simulink model "Bilanciamento_MPC"  (R2026b)
settings: Solver=FixedStepDiscrete  StartTime=0  StopTime=sl.t_fine  FixedStep=sl.Ts_integrazione
PostLoadFcn:
  | addpath(genpath(fileparts(fileparts(get_param('Bilanciamento_MPC', 'FileName')))));
  | if ~evalin('base', 'exist(''sl'', ''var'')')
  |     assignin('base', 'sl', init_simulink());
  | end
InitFcn:
  | addpath(genpath(fileparts(fileparts(get_param('Bilanciamento_MPC', 'FileName')))));
  | if ~evalin('base', 'exist(''sl'', ''var'')')
  |     assignin('base', 'sl', init_simulink());
  | end
undefined symbols (not defined in the file or in its folder): sl
libraries: simulink x2
settings Model: Creator=Acer  LastModifiedBy=Acer

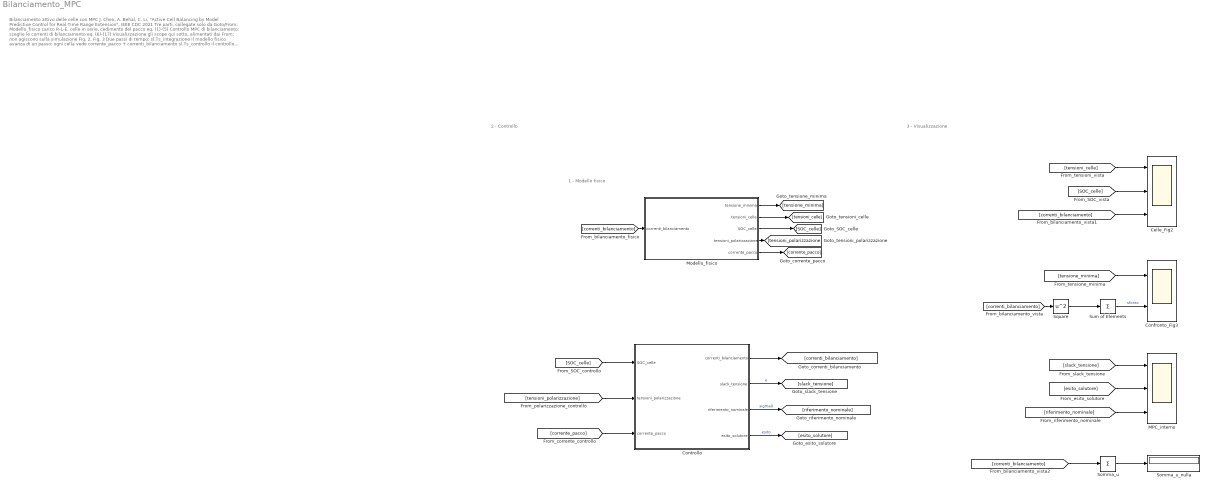
== system Bilanciamento_MPC ==
  note: Bilanciamento attivo delle celle con MPC
      | J. Chen, A. Behal, C. Li, "Active Cell Balancing by Model Predictive Control for Real Time Range Extension", IEEE CDC 2021
      |
      | Tre parti, collegate solo da Goto/From:
      |    Modello_fisico     carico R-L-E, celle in serie, cedimento del pacco             eq. (1)-(5)
      |    Controllo          MPC di bilanciamento: sceglie le correnti di bilanciamento    eq. (6)-(17)
      |    Visualizzazione    gli scope qui sotto, alimentati dai From: non agiscono sulla simulazione   Fig. 2, Fig. 3
      |
      | Due passi di tempo:
      |    sl.Ts_integrazione   il modello fisico avanza di un passo: ogni cella vede corrente_pacco + correnti_bilanciamento
      |    sl.Ts_controllo      il controllo campiona corrente_pacco, SOC_celle e tensioni_polarizzazione e sceglie correnti_bilanciamento,
      |                         che restano costanti fino al passo di controllo successivo
      | La simulazione si ferma quando una cella scende sotto y_min.
      |
      | Parametri nella struct 'sl' (avvio_simulink.m).  sl.tipo: 1 = J_t   2 = J_m   3 = J_Delta.  Confronto dei quattro casi: main_simulink.m
  note: 1 - Modello fisico
  note: 2 - Controllo
  note: 3 - Visualizzazione
  Celle_Fig2 : Scope  NumInputPorts=3
      settings: AttributesFormatString=Fig. 2: y, s, u  ActiveDisplayString=3  Title=Corrente di bilanciamento u^n [A]  ActiveDisplayYMinimum=-2.4917702044223984  ActiveDisplayYMaximum=2.42593183980159
  Confronto_Fig3 : Scope  NumInputPorts=2
      settings: AttributesFormatString=Fig. 3: min y, sforzo  Title=Sforzo di bilanciamento e_k = u_k'u_k [A^2]  ActiveDisplayYMinimum=0.52817346836693146  ActiveDisplayYMaximum=4.5629080222727767  DataLoggingVariableName=ScopeData2
  Controllo : Subsystem
      settings: AttributesFormatString=MPC: problema (6) risolto\ncome QP (Remark 3)
  MPC_interno : Scope  NumInputPorts=3
      settings: AttributesFormatString=slack e, esito, sigma0  ActiveDisplayString=3  Title=Riferimento della cella nominale sigma0, eq. (7): una linea per passo dell'orizzonte  ActiveDisplayYMinimum=-0.5240999999999999  ActiveDisplayYMaximum=4.7169
  Modello_fisico : Subsystem
      settings: AttributesFormatString=carico, celle, cedimento\neq. (1)-(5)
  Somma_u : Sum  Inputs=+
      settings: AttributesFormatString=eq. (6f)
  Somma_u_nulla : Display
      settings: AttributesFormatString=deve restare 0
  Square : Math  Operator=square
  Sum of Elements : Sum  Inputs=+
  wires:
  [correnti_bilanciamento] -> Square/1
  Square/1 -> Sum of Elements/1
  [correnti_bilanciamento] -> Somma_u/1
  [correnti_bilanciamento] -> Celle_Fig2/3
  [riferimento_nominale] -> MPC_interno/3
  [esito_solutore] -> MPC_interno/2
  [SOC_celle] -> Celle_Fig2/2
  [slack_tensione] -> MPC_interno/1
  [tensioni_celle] -> Celle_Fig2/1
  Sum of Elements/1 -> Confronto_Fig3/2  "sforzo"
  [tensione_minima] -> Confronto_Fig3/1
  Somma_u/1 -> Somma_u_nulla/1
  Controllo/4(esito_solutore) -> [esito_solutore]  "esito"
  Controllo/3(riferimento_nominale) -> [riferimento_nominale]  "sigma0"
  Controllo/2(slack_tensione) -> [slack_tensione]  "e"
  Controllo/1(correnti_bilanciamento) -> [correnti_bilanciamento]
  Modello_fisico/5(corrente_pacco) -> [corrente_pacco]
  Modello_fisico/4(tensioni_polarizzazione) -> [tensioni_polarizzazione]
  Modello_fisico/3(SOC_celle) -> [SOC_celle]
  Modello_fisico/2(tensioni_celle) -> [tensioni_celle]
  Modello_fisico/1(tensione_minima) -> [tensione_minima]
  [corrente_pacco] -> Controllo/3(corrente_pacco)
  [tensioni_polarizzazione] -> Controllo/2(tensioni_polarizzazione)
  [SOC_celle] -> Controllo/1(SOC_celle)
  [correnti_bilanciamento] -> Modello_fisico/1(correnti_bilanciamento)

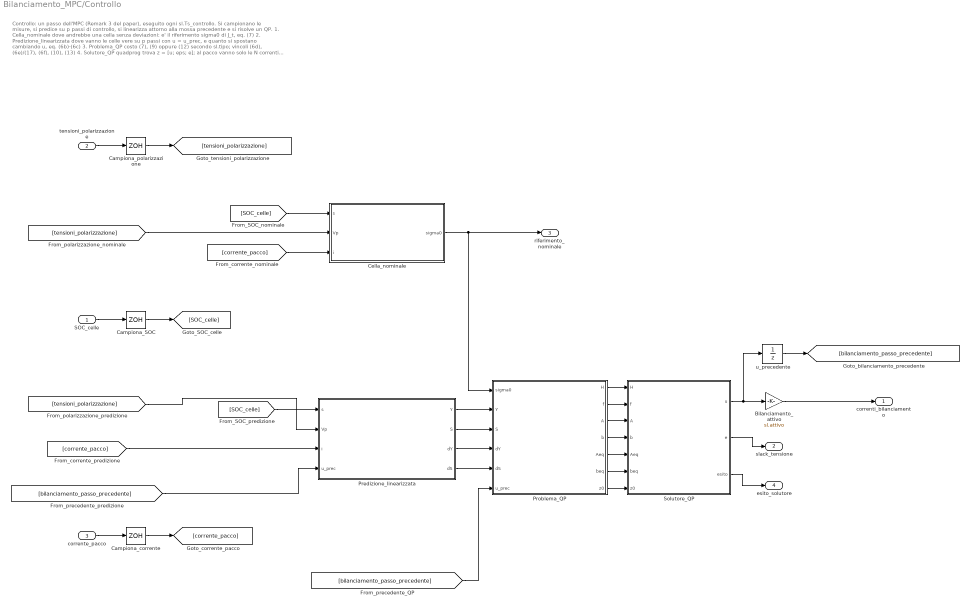
== system Bilanciamento_MPC/Controllo ==
  note: Controllo: un passo dell'MPC (Remark 3 del paper), eseguito ogni sl.Ts_controllo. Si campionano le misure, si predice su p passi di controllo,
      | si linearizza attorno alla mossa precedente e si risolve un QP.
      |
      | 1. Cella_nominale            dove andrebbe una cella senza deviazioni: e' il riferimento sigma0 di J_t, eq. (7)
      | 2. Predizione_linearizzata   dove vanno le celle vere su p passi con u = u_prec, e quanto si spostano cambiando u, eq. (6b)-(6c)
      | 3. Problema_QP               costo (7), (9) oppure (12) secondo sl.tipo; vincoli (6d), (6e)/(17), (6f), (10), (13)
      | 4. Solutore_QP               quadprog trova z = [u; eps; e]; al pacco vanno solo le N correnti u (orizzonte mobile)
      | 5. Bilanciamento_attivo      guadagno sl.attivo: con 0 il pacco lavora senza bilanciamento
      |
      | Doppio clic su un blocco per leggerne il codice; il calcolo vero e' nel file qp_*.m indicato nel commento.
  SOC_celle : Inport
  tensioni_polarizzazione : Inport  Port=2
  corrente_pacco : Inport  Port=3
  Bilanciamento_attivo : Gain  Gain=sl.attivo
      settings: AttributesFormatString=sl.attivo: 0 o 1
  Campiona_SOC : ZeroOrderHold  SampleTime=sl.Ts_controllo
      settings: AttributesFormatString=ogni Ts_controllo
  Campiona_corrente : ZeroOrderHold  SampleTime=sl.Ts_controllo
      settings: AttributesFormatString=ogni Ts_controllo
  Campiona_polarizzazione : ZeroOrderHold  SampleTime=sl.Ts_controllo
      settings: AttributesFormatString=ogni Ts_controllo
  Cella_nominale : MATLAB Function  TreatAsAtomicUnit=on
      settings: AttributesFormatString=eq. (7): riferimento sigma0
  Predizione_linearizzata : MATLAB Function  TreatAsAtomicUnit=on
      settings: AttributesFormatString=eq. (6b)-(6c), Remark 3
  Problema_QP : MATLAB Function  TreatAsAtomicUnit=on
      settings: AttributesFormatString=costo (7)/(9)/(12) e vincoli
  Solutore_QP : MATLAB Function  TreatAsAtomicUnit=on
      settings: AttributesFormatString=quadprog
  u_precedente : UnitDelay  InitialCondition=zeros(sl.N, 1)  SampleTime=sl.Ts_controllo
      settings: AttributesFormatString=u_(k-1)
  correnti_bilanciamento : Outport
  slack_tensione : Outport  Port=2
  riferimento_nominale : Outport  Port=3
  esito_solutore : Outport  Port=4
  wires:
  corrente_pacco/1 -> Campiona_corrente/1
  tensioni_polarizzazione/1 -> Campiona_polarizzazione/1
  SOC_celle/1 -> Campiona_SOC/1
  [corrente_pacco] -> Predizione_linearizzata/3(i)
  [tensioni_polarizzazione] -> Predizione_linearizzata/2(Vp)
  [SOC_celle] -> Predizione_linearizzata/1(s)
  [corrente_pacco] -> Cella_nominale/3(i)
  [tensioni_polarizzazione] -> Cella_nominale/2(Vp)
  [SOC_celle] -> Cella_nominale/1(s)
  Cella_nominale/1(sigma0) -> riferimento_nominale/1, Problema_QP/1(sigma0)
  Predizione_linearizzata/1(Y) -> Problema_QP/2(Y)
  Predizione_linearizzata/2(S) -> Problema_QP/3(S)
  Predizione_linearizzata/3(dY) -> Problema_QP/4(dY)
  Predizione_linearizzata/4(dS) -> Problema_QP/5(dS)
  Problema_QP/1(H) -> Solutore_QP/1(H)
  Problema_QP/2(f) -> Solutore_QP/2(f)
  Problema_QP/3(A) -> Solutore_QP/3(A)
  Problema_QP/4(b) -> Solutore_QP/4(b)
  Problema_QP/5(Aeq) -> Solutore_QP/5(Aeq)
  Problema_QP/6(beq) -> Solutore_QP/6(beq)
  Problema_QP/7(z0) -> Solutore_QP/7(z0)
  Solutore_QP/2(e) -> slack_tensione/1
  Solutore_QP/3(esito) -> esito_solutore/1
  [bilanciamento_passo_precedente] -> Predizione_linearizzata/4(u_prec)
  [bilanciamento_passo_precedente] -> Problema_QP/6(u_prec)
  u_precedente/1 -> [bilanciamento_passo_precedente]
  Bilanciamento_attivo/1 -> correnti_bilanciamento/1
  Solutore_QP/1(u) -> Bilanciamento_attivo/1, u_precedente/1
  Campiona_corrente/1 -> [corrente_pacco]
  Campiona_polarizzazione/1 -> [tensioni_polarizzazione]
  Campiona_SOC/1 -> [SOC_celle]

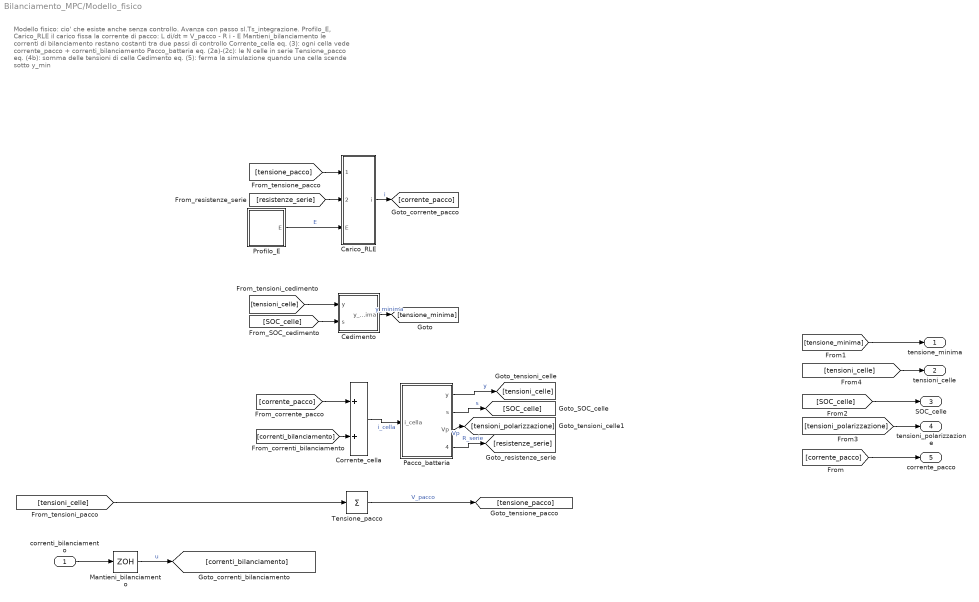
== system Bilanciamento_MPC/Modello_fisico ==
  note: Modello fisico: cio' che esiste anche senza controllo. Avanza con passo sl.Ts_integrazione.
      |
      |    Profilo_E, Carico_RLE   il carico fissa la corrente di pacco:  L di/dt = V_pacco - R i - E
      |    Mantieni_bilanciamento  le correnti di bilanciamento restano costanti tra due passi di controllo
      |    Corrente_cella          eq. (3): ogni cella vede corrente_pacco + correnti_bilanciamento
      |    Pacco_batteria          eq. (2a)-(2c): le N celle in serie
      |    Tensione_pacco          eq. (4b): somma delle tensioni di cella
      |    Cedimento               eq. (5): ferma la simulazione quando una cella scende sotto y_min
  correnti_bilanciamento : Inport
  Carico_RLE : Subsystem
      settings: AttributesFormatString=L di/dt = V_pacco - R i - E
  Cedimento : Subsystem
      settings: AttributesFormatString=eq. (5): y^n >= y_min
  Corrente_cella : Sum
      settings: AttributesFormatString=eq. (3): i + u^n
  Mantieni_bilanciamento : ZeroOrderHold  SampleTime=sl.Ts_integrazione
      settings: AttributesFormatString=costante tra due passi\ndi controllo
  Pacco_batteria : Subsystem
      settings: AttributesFormatString=eq. (2a)-(2c), (4a)
  Profilo_E : Subsystem
      settings: AttributesFormatString=f.e.m. del carico E(t)
  Tensione_pacco : Sum  Inputs=+
      settings: AttributesFormatString=eq. (4b)
  tensione_minima : Outport
  tensioni_celle : Outport  Port=2
  SOC_celle : Outport  Port=3
  tensioni_polarizzazione : Outport  Port=4
  corrente_pacco : Outport  Port=5
  wires:
  correnti_bilanciamento/1 -> Mantieni_bilanciamento/1
  [SOC_celle] -> Cedimento/2(s)
  [tensioni_celle] -> Tensione_pacco/1
  Pacco_batteria/1(y) -> [tensioni_celle]  "y"
  [tensioni_celle] -> Cedimento/1(y)
  [correnti_bilanciamento] -> Corrente_cella/2
  [tensione_pacco] -> Carico_RLE/1(V_pacco)
  Pacco_batteria/2(s) -> [SOC_celle]  "s"
  Tensione_pacco/1 -> [tensione_pacco]  "V_pacco"
  [resistenze_serie] -> Carico_RLE/2(R_serie)
  Pacco_batteria/4(R_serie) -> [resistenze_serie]  "R_serie"
  Profilo_E/1(E) -> Carico_RLE/3(E)  "E"
  Corrente_cella/1 -> Pacco_batteria/1(i_cella)  "i_cella"
  Carico_RLE/1(i) -> [corrente_pacco]  "i"
  [corrente_pacco] -> Corrente_cella/1
  Mantieni_bilanciamento/1 -> [correnti_bilanciamento]  "u"
  [corrente_pacco] -> corrente_pacco/1
  Cedimento/1(y_minima) -> [tensione_minima]  "y_minima"
  [tensione_minima] -> tensione_minima/1
  [SOC_celle] -> SOC_celle/1
  Pacco_batteria/3(Vp) -> [tensioni_polarizzazione]  "Vp"
  [tensioni_polarizzazione] -> tensioni_polarizzazione/1
  [tensioni_celle] -> tensioni_celle/1

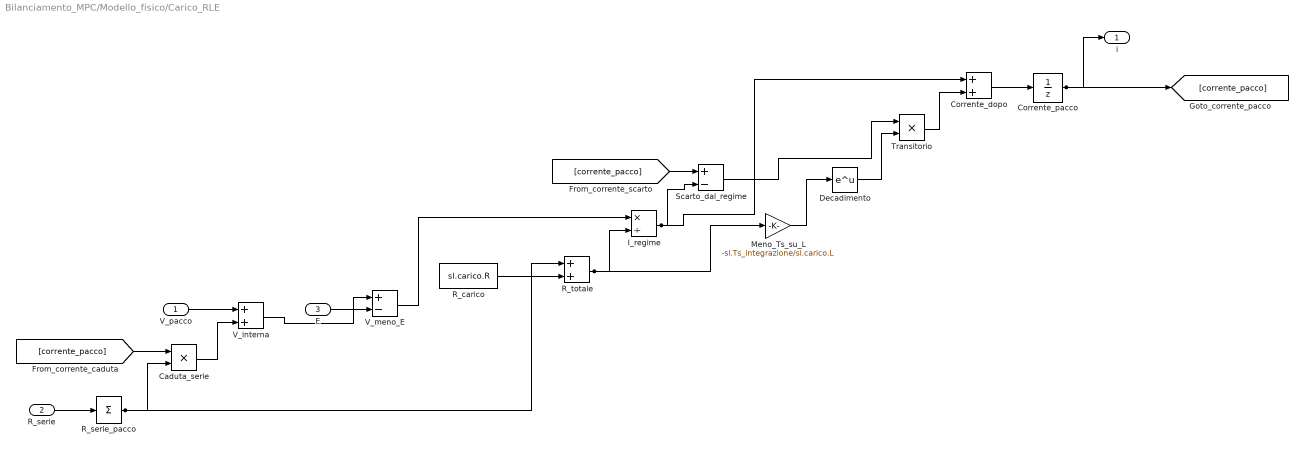
== system Bilanciamento_MPC/Modello_fisico/Carico_RLE ==
  V_pacco : Inport
  R_serie : Inport  Port=2
  E : Inport  Port=3
  Caduta_serie : Product  Inputs=**
  Corrente_dopo : Sum
  Corrente_pacco : UnitDelay  InitialCondition=sl.i_iniziale  SampleTime=sl.Ts_integrazione
      settings: AttributesFormatString=stato i
  Decadimento : Math
      settings: AttributesFormatString=exp(-Ts_integrazione*R_totale/L)
  I_regime : Product  Inputs=*/
      settings: AttributesFormatString=(V_interna - E) / R_totale
  Meno_Ts_su_L : Gain  Gain=-sl.Ts_integrazione/sl.carico.L
  R_carico : Constant  Value=sl.carico.R  SampleTime=sl.Ts_integrazione
  R_serie_pacco : Sum  Inputs=+
  R_totale : Sum
  Scarto_dal_regime : Sum  Inputs=+-
  Transitorio : Product  Inputs=**
  V_interna : Sum
      settings: AttributesFormatString=tensione del pacco a i = 0
  V_meno_E : Sum  Inputs=+-
  i : Outport
  wires:
  [corrente_pacco] -> Scarto_dal_regime/1
  [corrente_pacco] -> Caduta_serie/1
  R_serie/1 -> R_serie_pacco/1
  R_serie_pacco/1 -> Caduta_serie/2, R_totale/1
  R_carico/1 -> R_totale/2
  Corrente_pacco/1 -> i/1, [corrente_pacco]
  V_pacco/1 -> V_interna/1
  Caduta_serie/1 -> V_interna/2
  V_interna/1 -> V_meno_E/1
  E/1 -> V_meno_E/2
  V_meno_E/1 -> I_regime/1
  R_totale/1 -> Meno_Ts_su_L/1, I_regime/2
  Meno_Ts_su_L/1 -> Decadimento/1
  I_regime/1 -> Corrente_dopo/1, Scarto_dal_regime/2
  Scarto_dal_regime/1 -> Transitorio/1
  Decadimento/1 -> Transitorio/2
  Transitorio/1 -> Corrente_dopo/2
  Corrente_dopo/1 -> Corrente_pacco/1

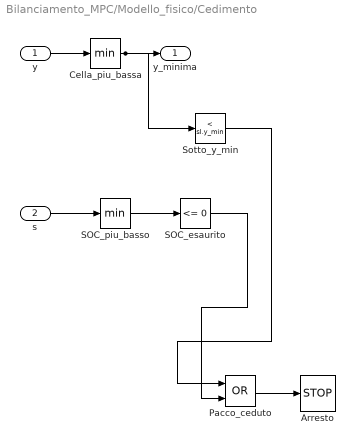
== system Bilanciamento_MPC/Modello_fisico/Cedimento ==
  y : Inport
  s : Inport  Port=2
  Arresto : Stop
  Cella_piu_bassa : MinMax
  Pacco_ceduto : Logic  Operator=OR  IconShape=distinctive  AllPortsSameDT=off  OutDataTypeStr=boolean
  SOC_esaurito : simulink/Logic and Bit Operations/Compare To Constant  relop=<=  const=0  OutDataTypeStr=boolean
  SOC_piu_basso : MinMax
  Sotto_y_min : simulink/Logic and Bit Operations/Compare To Constant  relop=<  const=sl.y_min  OutDataTypeStr=boolean
  y_minima : Outport
  wires:
  y/1 -> Cella_piu_bassa/1
  s/1 -> SOC_piu_basso/1
  Cella_piu_bassa/1 -> y_minima/1, Sotto_y_min/1
  SOC_piu_basso/1 -> SOC_esaurito/1
  Sotto_y_min/1 -> Pacco_ceduto/1
  SOC_esaurito/1 -> Pacco_ceduto/2
  Pacco_ceduto/1 -> Arresto/1

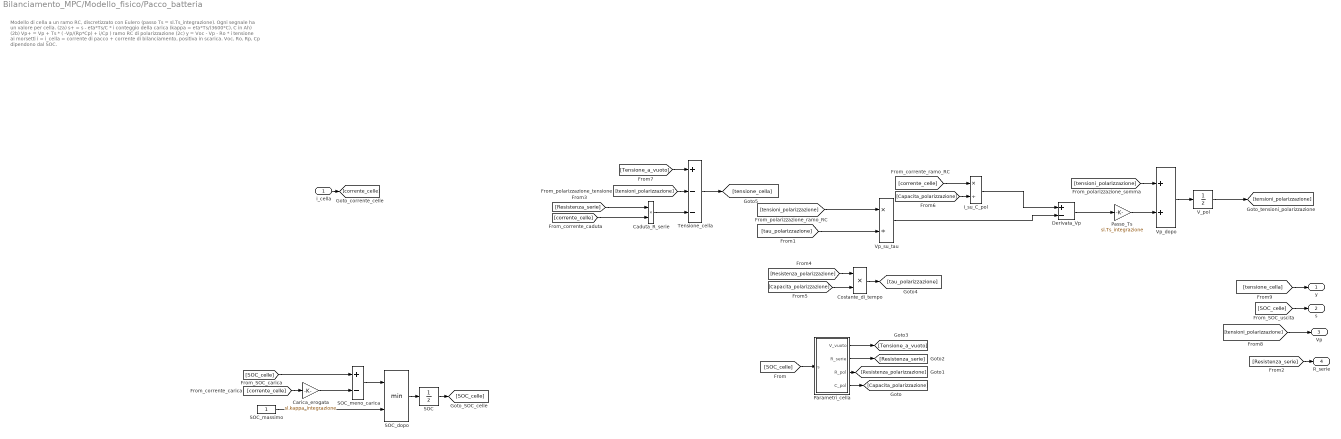
== system Bilanciamento_MPC/Modello_fisico/Pacco_batteria ==
  note: Modello di cella a un ramo RC, discretizzato con Eulero (passo Ts = sl.Ts_integrazione). Ogni segnale ha un valore per cella.
      |
      | (2a)   s+   =  s  -  eta*Ts/C * i                        conteggio della carica (kappa = eta*Ts/(3600*C), C in Ah)
      | (2b)   Vp+  =  Vp  +  Ts * ( -Vp/(Rp*Cp)  +  i/Cp )      ramo RC di polarizzazione
      | (2c)   y    =  Voc  -  Vp  -  Ro * i                     tensione ai morsetti
      |
      | i = i_cella = corrente di pacco + corrente di bilanciamento, positiva in scarica.  Voc, Ro, Rp, Cp dipendono dal SOC.
  i_cella : Inport
  Caduta_R_serie : Product  Inputs=**
  Carica_erogata : Gain  Gain=sl.kappa_integrazione
      settings: AttributesFormatString=kappa * i
  Costante_di_tempo : Product  Inputs=**
  Derivata_Vp : Sum  Inputs=+-
  I_su_C_pol : Product  Inputs=*/
  Parametri_cella : Subsystem
      settings: AttributesFormatString=V_oc, R_o, R_p, C_p(SOC)
  Passo_Ts : Gain  Gain=sl.Ts_integrazione
  SOC : UnitDelay  InitialCondition=sl.SOC_iniziale  SampleTime=sl.Ts_integrazione
      settings: AttributesFormatString=stato s
  SOC_dopo : MinMax  Inputs=2
      settings: AttributesFormatString=eq. (2a)
  SOC_massimo : Constant  SampleTime=sl.Ts_integrazione
  SOC_meno_carica : Sum  Inputs=+-
  Tensione_cella : Sum  Inputs=+--
      settings: AttributesFormatString=eq. (2c)
  V_pol : UnitDelay  InitialCondition=sl.Vp_iniziale  SampleTime=sl.Ts_integrazione
      settings: AttributesFormatString=stato V_p
  Vp_dopo : Sum
      settings: AttributesFormatString=eq. (2b)
  Vp_su_tau : Product  Inputs=*/
  y : Outport
  s : Outport  Port=2
  Vp : Outport  Port=3
  R_serie : Outport  Port=4
  wires:
  i_cella/1 -> [corrente_celle]
  [tensioni_polarizzazione] -> Vp_dopo/1
  [tensioni_polarizzazione] -> Vp_su_tau/1
  [tensioni_polarizzazione] -> Tensione_cella/2
  [SOC_celle] -> s/1
  [SOC_celle] -> SOC_meno_carica/1
  [corrente_celle] -> I_su_C_pol/1
  [corrente_celle] -> Carica_erogata/1
  [corrente_celle] -> Caduta_R_serie/2
  Vp_dopo/1 -> V_pol/1
  Passo_Ts/1 -> Vp_dopo/2
  Derivata_Vp/1 -> Passo_Ts/1
  Vp_su_tau/1 -> Derivata_Vp/2
  I_su_C_pol/1 -> Derivata_Vp/1
  SOC_dopo/1 -> SOC/1
  SOC_massimo/1 -> SOC_dopo/2
  SOC_meno_carica/1 -> SOC_dopo/1
  Carica_erogata/1 -> SOC_meno_carica/2
  Caduta_R_serie/1 -> Tensione_cella/3
  V_pol/1 -> [tensioni_polarizzazione]
  SOC/1 -> [SOC_celle]
  [SOC_celle] -> Parametri_cella/1(s)
  [Resistenza_serie] -> R_serie/1
  [Resistenza_serie] -> Caduta_R_serie/1
  Parametri_cella/2(R_serie) -> [Resistenza_serie]
  [Resistenza_polarizzazione] -> Costante_di_tempo/1
  Parametri_cella/3(R_pol) -> [Resistenza_polarizzazione]
  Parametri_cella/4(C_pol) -> [Capacita_polarizzazione]
  [Capacita_polarizzazione] -> Costante_di_tempo/2
  [Capacita_polarizzazione] -> I_su_C_pol/2
  [Tensione_a_vuoto] -> Tensione_cella/1
  Parametri_cella/1(V_vuoto) -> [Tensione_a_vuoto]
  Costante_di_tempo/1 -> [tau_polarizzazione]
  [tau_polarizzazione] -> Vp_su_tau/2
  [tensioni_polarizzazione] -> Vp/1
  [tensione_cella] -> y/1
  Tensione_cella/1 -> [tensione_cella]

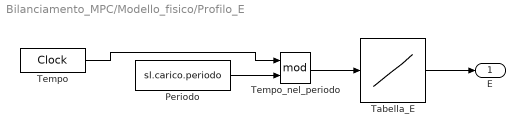
== system Bilanciamento_MPC/Modello_fisico/Profilo_E ==
  Periodo : Constant  Value=sl.carico.periodo  SampleTime=sl.Ts_integrazione
  Tabella_E : Lookup_n-D  NumberOfTableDimensions=1  BreakpointsForDimension1=sl.carico.t_E  Table=sl.carico.E  ExtrapMethod=Clip  InternalRulePriority=Speed  RndMeth=Simplest
  Tempo : DigitalClock  SampleTime=sl.Ts_integrazione
  Tempo_nel_periodo : Math  Operator=mod
  E : Outport
  wires:
  Tempo/1 -> Tempo_nel_periodo/1
  Periodo/1 -> Tempo_nel_periodo/2
  Tempo_nel_periodo/1 -> Tabella_E/1
  Tabella_E/1 -> E/1

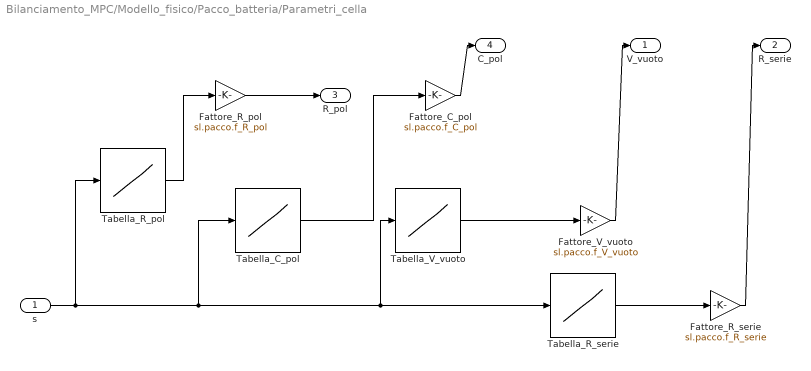
== system Bilanciamento_MPC/Modello_fisico/Pacco_batteria/Parametri_cella ==
  s : Inport
  Fattore_C_pol : Gain  Gain=sl.pacco.f_C_pol
  Fattore_R_pol : Gain  Gain=sl.pacco.f_R_pol
  Fattore_R_serie : Gain  Gain=sl.pacco.f_R_serie
  Fattore_V_vuoto : Gain  Gain=sl.pacco.f_V_vuoto
  Tabella_C_pol : Lookup_n-D  NumberOfTableDimensions=1  BreakpointsForDimension1=sl.pacco.tabella_SOC  Table=sl.pacco.tabella_C_pol  ExtrapMethod=Clip  InternalRulePriority=Speed  RndMeth=Simplest
  Tabella_R_pol : Lookup_n-D  NumberOfTableDimensions=1  BreakpointsForDimension1=sl.pacco.tabella_SOC  Table=sl.pacco.tabella_R_pol  ExtrapMethod=Clip  InternalRulePriority=Speed  RndMeth=Simplest
  Tabella_R_serie : Lookup_n-D  NumberOfTableDimensions=1  BreakpointsForDimension1=sl.pacco.tabella_SOC  Table=sl.pacco.tabella_R_serie  ExtrapMethod=Clip  InternalRulePriority=Speed  RndMeth=Simplest
  Tabella_V_vuoto : Lookup_n-D  NumberOfTableDimensions=1  BreakpointsForDimension1=sl.pacco.tabella_SOC  Table=sl.pacco.tabella_V_vuoto  ExtrapMethod=Clip  InternalRulePriority=Speed  RndMeth=Simplest
  V_vuoto : Outport
  R_serie : Outport  Port=2
  R_pol : Outport  Port=3
  C_pol : Outport  Port=4
  wires:
  s/1 -> Tabella_R_serie/1, Tabella_V_vuoto/1, Tabella_C_pol/1, Tabella_R_pol/1
  Tabella_V_vuoto/1 -> Fattore_V_vuoto/1
  Tabella_R_serie/1 -> Fattore_R_serie/1
  Tabella_R_pol/1 -> Fattore_R_pol/1
  Tabella_C_pol/1 -> Fattore_C_pol/1
  Fattore_V_vuoto/1 -> V_vuoto/1
  Fattore_R_serie/1 -> R_serie/1
  Fattore_R_pol/1 -> R_pol/1
  Fattore_C_pol/1 -> C_pol/1

== matlab function Bilanciamento_MPC/Controllo/Predizione_linearizzata ==
  data: s input; Y output; Vp input; i input; u_prec input; S output; dY output; dS output; sl parameter
function [Y, S, dY, dS] = Predizione_linearizzata(s, Vp, i, u_prec, sl)
% Modello di predizione, eq. (6b)-(6c), linearizzato come nel Remark 3.
%
% Integra le celle per p passi di controllo con la corrente i + u_prec tenuta costante e
% calcola le derivate rispetto a u:
%   y_{k+j}(u) ~= Y(j,:) + dY(j,:) .* (u - u_prec)
%   s_{k+j}(u) ~= S(j,:) + dS(j,:) .* (u - u_prec)
% Y, S, dY, dS sono p x N: riga j <-> istante k+j, colonna n <-> cella n.
%
% Codice: qp_predizione.m

[Y, S, dY, dS] = qp_predizione(sl.pacco, s, Vp, i + u_prec, sl.p, sl.Ts_controllo);

== matlab function Bilanciamento_MPC/Controllo/Cella_nominale ==
  data: s input; sigma0 output; Vp input; i input; sl parameter
function sigma0 = Cella_nominale(s, Vp, i, sl)
% Riferimento per J_t, eq. (7) del paper.
%
% La cella nominale (parametri senza deviazione) parte dalla media degli stati
% del pacco e viene integrata su p passi con la sola corrente di pacco i.
% sigma0 e' p x 1: riga j <-> istante k+j.
%
% Codice: qp_cella_nominale.m

sigma0 = qp_cella_nominale(sl, s, Vp, i);

== matlab function Bilanciamento_MPC/Controllo/Problema_QP ==
  data: sigma0 input; H output; Y input; S input; dY input; dS input; u_prec input; f output; A output; b output; Aeq output; beq output; z0 output; sl parameter
function [H, f, A, b, Aeq, beq, z0] = Problema_QP(sigma0, Y, S, dY, dS, u_prec, sl)
% Il problema (6) del paper scritto come QP nelle incognite z = [u; eps; e]:
%
%   min 1/2*z'*H*z + f'*z    con  A*z <= b,  Aeq*z = beq
%
%   H, f      costo: (7) per Jt, (9) per Jm, (12) per Jdelta, piu' u'*R*u e W*e^2
%   A, b      (6e) rilassata come in (17), (10)/(13) sulle eps, limiti (6d)
%   Aeq, beq  (6f): somma delle u nulla
%   z0        punto di partenza: la mossa del passo precedente
%
% Codice: qp_problema.m

[H, f, A, b, Aeq, beq, z0] = qp_problema(sl, sigma0, Y, S, dY, dS, u_prec);

== matlab function Bilanciamento_MPC/Controllo/Solutore_QP ==
  data: H input; u output; f input; A input; b input; Aeq input; beq input; z0 input; e output; esito output; sl parameter
function [u, e, esito] = Solutore_QP(H, f, A, b, Aeq, beq, z0, sl)
% Risolve il QP con quadprog e applica solo le correnti di bilanciamento u.
%
%   u      prime N componenti di z: le correnti da applicare al passo k
%   e      ultima componente di z: slack del vincolo di tensione, eq. (17)
%   esito  exitflag di quadprog (1 = soluzione trovata)
%
% Codice: qp_solutore.m (eseguito da MATLAB, non compilato)

coder.extrinsic('qp_solutore');

z     = z0;
esito = 0;
[z, esito] = qp_solutore(H, f, A, b, Aeq, beq, z0);

u = z(1:sl.N);
e = z(end);
